simulink model "highpassFilter"  (R2020a)
settings: Solver=VariableStepAuto  StartTime=0.0  StopTime=tStop  MaxStep=dt  RelTol=1e-3
settings Model: Creator=DELL  LastModifiedBy=DELL

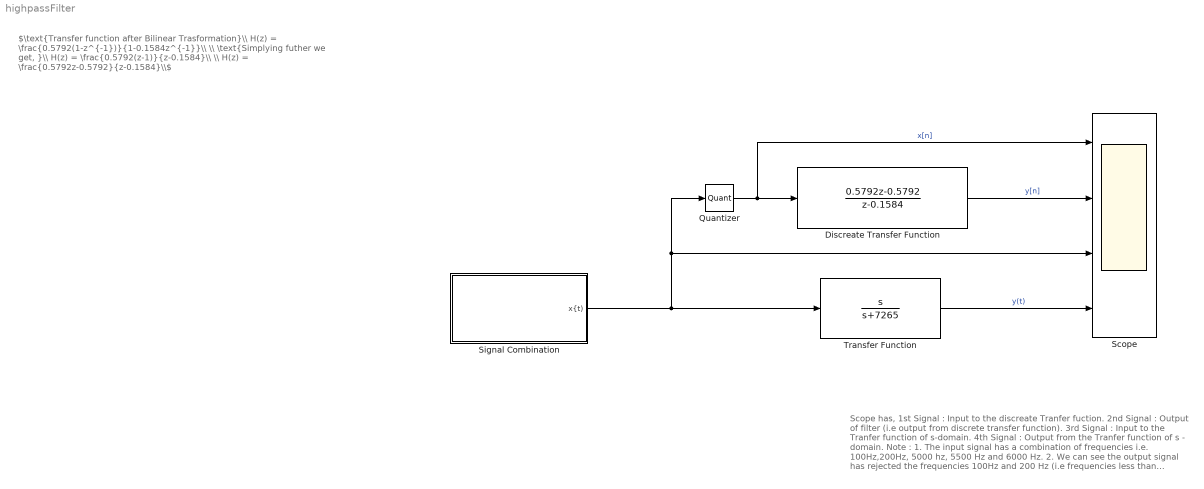
== system highpassFilter ==
  note: Scope has,
      | 1st Signal  : Input to the discreate Tranfer fuction.
      | 2nd Signal : Output of filter (i.e output from discrete transfer function).
      | 3rd Signal  : Input to the Tranfer function of s-domain.
      | 4th Signal  : Output from the Tranfer function of s - domain.
      |
      | Note :
      |
      | 1. The input signal has a combination of frequencies i.e. 100Hz,200Hz,
      | 5000 hz, 5500 Hz and 6000 Hz.
      | 2. We can see the output signal has rejected the frequencies 100Hz
      | and 200 Hz (i.e frequencies less than 1000Hz), also the frequencies
      | 5000 Hz. 550Hz and 6000 Hz are passed hence realising a High Pass filter.
  note: $\text{Transfer function after Bilinear Trasformation}\\ H(z) = \frac{0.5792(1-z^{-1})}{1-0.1584z^{-1}}\\ \\ \text{Simplying futher we get, }\\ H(z) = \frac{0.5792(z-1)}{z-0.1584}\\ \\ H(z) = \frac{0.5792z-0.5792}{z-0.1584}\\$
  Discreate Transfer Function : DiscreteTransferFcn  Numerator=[0.5792 -0.5792]  Denominator=[1 -0.1584]
  Quantizer : Quantizer
  Scope : Scope  NumInputPorts=4
  Signal Combination : Subsystem  mask{Amp1=5, freq1=100, Amp2=4, freq2=200, Amp3=2, freq3=5000, Amp4=1, freq4=5500, Amp5=1, freq5=6000}
      mask prompts: Amp1 "Amplitude"; freq1 "Frequency"; Amp2 "Amplitude"; freq2 "Frequency"; Amp3 "Amplitude"; freq3 "Frequency"; Amp4 "Amplitude"; freq4 "Frequency"; Amp5 "Amplitude"; freq5 "Frequency"
      mask DialogControl DescGroupVar Prompt: Signal Combination
      mask DialogControl Container3 Prompt: Signal 1
      mask DialogControl Container4 Prompt: Signal 2
      mask DialogControl Container5 Prompt: Signal 3
      mask DialogControl Container6 Prompt: Signal 4
      mask DialogControl Container7 Prompt: Signal 5
  Transfer Function : TransferFcn  Numerator=[1 0]  Denominator=[1 7265]
  wires:
  Quantizer/1 -> Discreate Transfer Function/1, Scope/1  "x[n]"
  Discreate Transfer Function/1 -> Scope/2  "y[n]"
  Transfer Function/1 -> Scope/4  "y(t)"
  Signal Combination/1("x{t)") -> Quantizer/1, Scope/3, Transfer Function/1

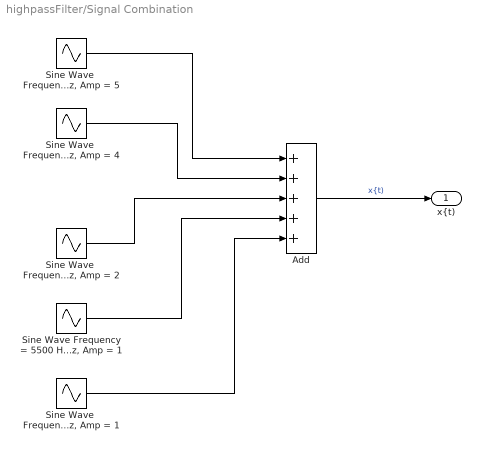
== system highpassFilter/Signal Combination ==
  Add : Sum  Inputs=+++++
  "Sine Wave  Frequency = 100 Hz, Amp = 5" : Sin  Amplitude=Amp1  Frequency=2*pi*freq1  SampleTime=0
  "Sine Wave  Frequency = 200 Hz, Amp = 4" : Sin  Amplitude=Amp2  Frequency=2*pi*freq2  SampleTime=0
  "Sine Wave  Frequency = 5000 Hz, Amp = 2" : Sin  Amplitude=Amp3  Frequency=2*pi*freq3  SampleTime=0
  "Sine Wave  Frequency = 6000 Hz, Amp = 1" : Sin  Amplitude=Amp5  Frequency=2*pi*freq5  SampleTime=0
  "Sine Wave Frequency = 5500 Hz, Amp = 1" : Sin  Amplitude=Amp3  Frequency=2*pi*freq4  SampleTime=0
  "x{t)" : Outport
  wires:
  "Sine Wave Frequency = 5500 Hz, Amp = 1"/1 -> Add/4
  "Sine Wave  Frequency = 100 Hz, Amp = 5"/1 -> Add/1
  "Sine Wave  Frequency = 5000 Hz, Amp = 2"/1 -> Add/3
  Add/1 -> "x{t)"/1  "x{t)"
  "Sine Wave  Frequency = 200 Hz, Amp = 4"/1 -> Add/2
  "Sine Wave  Frequency = 6000 Hz, Amp = 1"/1 -> Add/5
